simulink model "a"  (R2018b)
settings: Solver=VariableStepAuto  StartTime=0.0  StopTime=100  RelTol=1e-3
settings Model: Creator=aycfink  LastModifiedBy=aycfink

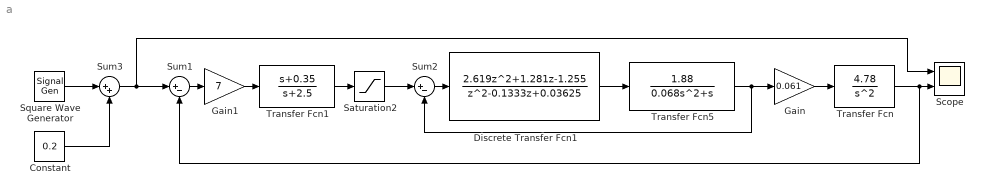
== system a ==
  Constant : Constant  Value=0.2
  Discrete Transfer Fcn1 : DiscreteTransferFcn  Numerator=[2.619 1.281 -1.255]  Denominator=[1 -0.1333 0.03625]  SampleTime=0.029012
  Gain : Gain  Gain=0.061
  Gain1 : Gain  Gain=7
  Saturation2 : Saturate  UpperLimit=0.7  LowerLimit=-0.7
  Scope : Scope  NumInputPorts=2
  Square Wave Generator : SignalGenerator  WaveForm=square  Amplitude=0.05  Frequency=0.2  Units=rad/sec
  Sum1 : Sum  Inputs=|+-
  Sum2 : Sum  Inputs=|+-
  Sum3 : Sum  Inputs=|++
  Transfer Fcn : TransferFcn  Numerator=[4.78]  Denominator=[1 0 0]
  Transfer Fcn1 : TransferFcn  Numerator=[1 0.35]  Denominator=[1 2.5]
  Transfer Fcn5 : TransferFcn  Numerator=[1.88]  Denominator=[0.068 1 0]
  wires:
  Saturation2/1 -> Sum2/1
  Transfer Fcn5/1 -> Sum2/2, Gain/1
  Discrete Transfer Fcn1/1 -> Transfer Fcn5/1
  Sum2/1 -> Discrete Transfer Fcn1/1
  Transfer Fcn1/1 -> Saturation2/1
  Gain/1 -> Transfer Fcn/1
  Transfer Fcn/1 -> Sum1/2, Scope/2
  Sum1/1 -> Gain1/1
  Gain1/1 -> Transfer Fcn1/1
  Square Wave Generator/1 -> Sum3/1
  Sum3/1 -> Scope/1, Sum1/1
  Constant/1 -> Sum3/2
